simulink model "Lab3"  (R2023b)
settings: Solver=VariableStepAuto  StartTime=0.0  StopTime=10000  MaxStep=0.1  RelTol=1e-3
values from neighbouring files (symbols this model uses):
  A = [-P1 0 -Gb;0 -n 0;0 P3 -P2]    [Parametri_Bergaman_model.m]
  B = [0 1/Vg;1/V1 0;0 0]    [Parametri_Bergaman_model.m]
  Gb = 81    [Parametri_Bergaman_model.m]
  Ib = 15    [Parametri_Bergaman_model.m]
  n = 5/54    (= 0.0925925925926)    [Parametri_Bergaman_model.m]
  p1 = P1    (= 0.003)    [Parametri_Bergaman_model.m]
  p2 = P2    (= 0.025)    [Parametri_Bergaman_model.m]
  p3 = P3    (= 1.3e-05)    [Parametri_Bergaman_model.m]
  Ub = 16.66667    [Parametri_Bergaman_model.m]
  V1 = 12    [Parametri_Bergaman_model.m]
  Vg = 126    [Parametri_Bergaman_model.m]
  x0lin = [9 0 0]'    [Parametri_Bergaman_model.m]
libraries: simulink x4
settings Model: Creator=Diego Regruto  LastModifiedBy=Diego Regruto

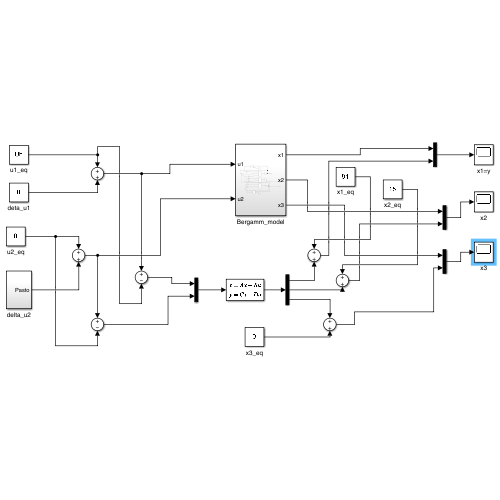
[thumbnail: Simulink's stored preview of the top-level diagram]
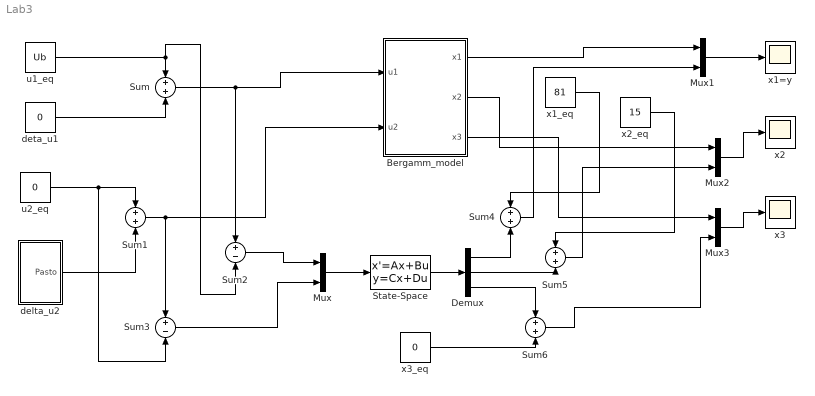
== system Lab3 ==
  Bergamm_model : Subsystem
  Demux : Demux  Outputs=3
  Mux{,1..3} (4 alike) : Mux  Inputs=2
  State-Space : StateSpace  A=A  B=B  C=eye(3,3)  D=zeros(3,2)  InitialCondition=x0lin
  Sum{,1,4..6} (5 alike) : Sum
  Sum2 : Sum  Inputs=+-
  Sum3 : Sum  Inputs=+-
  delta_u2 : Subsystem
  deta_u1 : Constant  Value=0
  u1_eq : Constant  Value=Ub
  u2_eq : Constant  Value=0
  x1=y : Scope
  x1_eq : Constant  Value=81
  x2 : Scope
  x2_eq : Constant  Value=15
  x3 : Scope
  x3_eq : Constant  Value=0
  wires:
  State-Space/1 -> Demux/1
  Mux/1 -> State-Space/1
  u1_eq/1 -> Sum2/2, Sum/1
  deta_u1/1 -> Sum/2
  Sum/1 -> Sum2/1, Bergamm_model/1(u1)
  u2_eq/1 -> Sum3/2, Sum1/1
  delta_u2/1(Pasto) -> Sum1/2
  Sum1/1 -> Sum3/1, Bergamm_model/2(u2)
  Sum2/1 -> Mux/1
  Sum3/1 -> Mux/2
  Demux/1 -> Sum4/2
  x1_eq/1 -> Sum4/1
  Demux/2 -> Sum5/2
  x2_eq/1 -> Sum5/1
  Demux/3 -> Sum6/1
  x3_eq/1 -> Sum6/2
  Bergamm_model/1(x1) -> Mux1/1
  Sum4/1 -> Mux1/2
  Mux1/1 -> x1=y/1
  Bergamm_model/2(x2) -> Mux2/1
  Mux2/1 -> x2/1
  Sum5/1 -> Mux2/2
  Bergamm_model/3(x3) -> Mux3/1
  Sum6/1 -> Mux3/2
  Mux3/1 -> x3/1

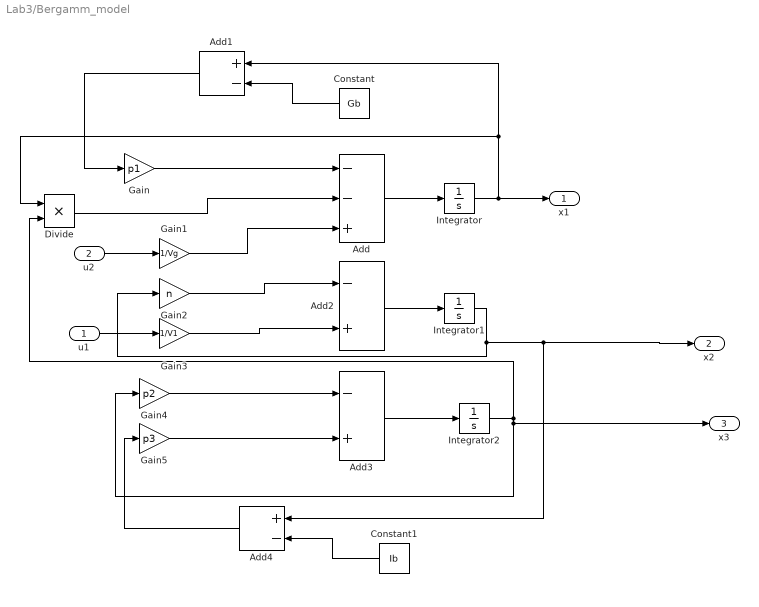
== system Lab3/Bergamm_model ==
  u1 : Inport
  u2 : Inport  Port=2
  Add : Sum  Inputs=--+
  Add1 : Sum  Inputs=+-
  Add2 : Sum  Inputs=-+
  Add3 : Sum  Inputs=-+
  Add4 : Sum  Inputs=+-
  Constant : Constant  Value=Gb
  Constant1 : Constant  Value=Ib
  Divide : Product  Inputs=**
  Gain : Gain  Gain=p1
  Gain1 : Gain  Gain=1/Vg
  Gain2 : Gain  Gain=n
  Gain3 : Gain  Gain=1/V1
  Gain4 : Gain  Gain=p2
  Gain5 : Gain  Gain=p3
  Integrator : Integrator  InitialCondition=81+9
  Integrator1 : Integrator  InitialCondition=15
  Integrator2 : Integrator
  x1 : Outport
  x2 : Outport  Port=2
  x3 : Outport  Port=3
  wires:
  Constant/1 -> Add1/2
  Add4/1 -> Gain5/1
  Divide/1 -> Add/2
  Integrator1/1 -> x2/1, Add4/1, Gain2/1
  Add3/1 -> Integrator2/1
  Constant1/1 -> Add4/2
  Integrator/1 -> x1/1, Divide/1, Add1/1
  Add/1 -> Integrator/1
  Gain4/1 -> Add3/1
  u2/1 -> Gain1/1
  Gain2/1 -> Add2/1
  u1/1 -> Gain3/1
  Add1/1 -> Gain/1
  Gain/1 -> Add/1
  Add2/1 -> Integrator1/1
  Gain3/1 -> Add2/2
  Integrator2/1 -> Divide/2, x3/1, Gain4/1
  Gain5/1 -> Add3/2
  Gain1/1 -> Add/3

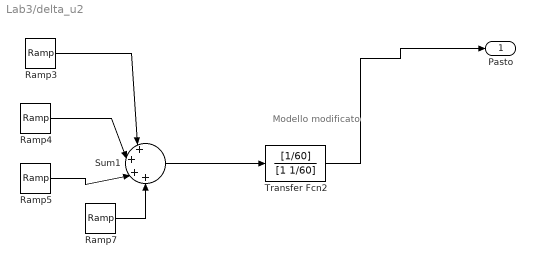
== system Lab3/delta_u2 ==
  note: Modello
      | modificato
  Ramp3 : simulink/Sources/Ramp  slope=12  start=0  InitialOutput=0
  Ramp4 : simulink/Sources/Ramp  slope=-12  start=30  InitialOutput=0
  Ramp5 : simulink/Sources/Ramp  slope=-12  start=90  InitialOutput=0
  Ramp7 : simulink/Sources/Ramp  slope=12  start=120  InitialOutput=0
  Sum1 : Sum  Inputs=|+|+|+|+  InputSameDT=on  SaturateOnIntegerOverflow=on  OutDataTypeStr=Inherit: Same as first input
  Transfer Fcn2 : TransferFcn  Numerator=[1/60]  Denominator=[1 1/60]
  Pasto : Outport
  wires:
  Ramp3/1 -> Sum1/1
  Ramp4/1 -> Sum1/2
  Ramp5/1 -> Sum1/3
  Ramp7/1 -> Sum1/4
  Sum1/1 -> Transfer Fcn2/1
  Transfer Fcn2/1 -> Pasto/1
